simulink model "elevator"  (R2021a)
settings: Solver=VariableStepAuto  StartTime=0.0  StopTime=10  RelTol=1e-3
settings Model: Creator=Oleg  LastModifiedBy=Oleg

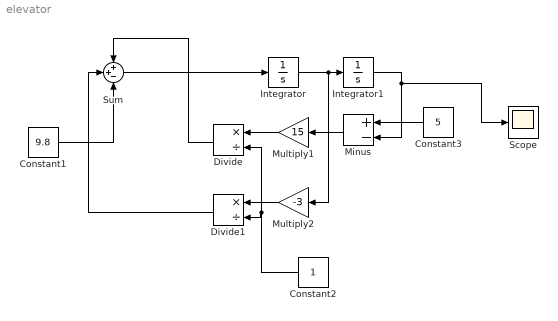
== system elevator ==
  Constant1 : Constant  Value=9.8
  Constant2 : Constant
  Constant3 : Constant  Value=5
  Divide : Product  Inputs=*/
  Divide1 : Product  Inputs=*/
  Integrator : Integrator
  Integrator1 : Integrator  InitialCondition=10
  Minus : Sum  Inputs=+-
  Multiply1 : Gain  Gain=15
  Multiply2 : Gain  Gain=-3
  Scope : Scope
  Sum : Sum  Inputs=++-
  wires:
  Integrator/1 -> Multiply2/1, Integrator1/1
  Sum/1 -> Integrator/1
  Minus/1 -> Multiply1/1
  Constant2/1 -> Divide1/2, Divide/2
  Multiply1/1 -> Divide/1
  Constant3/1 -> Minus/1
  Integrator1/1 -> Scope/1, Minus/2
  Multiply2/1 -> Divide1/1
  Divide1/1 -> Sum/2
  Divide/1 -> Sum/1
  Constant1/1 -> Sum/3
